simulink model "BugE_v0_40_MAS"  (R2015b)
settings: Solver=FixedStepDiscrete  StartTime=0.0  StopTime=inf  FixedStep=sample_time  RelTol=1e-3
values from neighbouring files (symbols this model uses):
  AB_diode_dV = 0.9    [main_sync.m]
  air_density = 1.225    [main_sync.m]
  bus_charger_Pmax = 1000    [main_sync.m]
  bus_load_Pmax_abs = 500    [main_sync.m]
  capInitVolt = capVmax*sqrt(capInitSoC)    [main_sync.m]
  cyc_kph = [cyc_kph(:,1), cyc_kph(:,2)*speed_max_limit/speed_max]    [main_sync.m]
  cyc_repeat = 0    [main_sync.m]
  ess1_init_soc = 1    [main_sync.m]
  ess1_soh = 1    [main_sync.m]
  ess2_init_soc = 1    [main_sync.m]
  ess2_soh = 1    [main_sync.m]
  ess3_init_soc = 1    [main_sync.m]
  ess3_soh = 1    [main_sync.m]
  ess4_init_soc = 1    [main_sync.m]
  ess4_soh = 1    [main_sync.m]
  ess5_init_soc = 1    [main_sync.m]
  ess5_soh = 1    [main_sync.m]
  gear_ratio = 6    [main_sync.m]
  loadpower = rawcsv(:,2)    [main_sync.m]
  loadtime = rawcsv(:,1)    [main_sync.m]
  lockSOCs = 0    [main_sync.m]
  max_brk_torque = 300    [main_sync.m]
  no_wheels = 3    [main_sync.m]
  period2 = max(loadtime)    [main_sync.m]
  PV_Pmax = 100    [main_sync.m]
  sample_time = 0.01    [main_sync.m]
  startup_seq_step_delay = 0.2    [main_sync.m]
  stop_option = 0    [main_sync.m]
  use_drive_cycle = 1    [main_sync.m]
  use_real_subs_loads = 1    [main_sync.m]
  vbus_max = 25    [main_sync.m]
  vbus_min = 17    [main_sync.m]
  vbus_safety_threshold = 2    [main_sync.m]
  vbus_threshold = 20    [main_sync.m]
  veh_CD = 0.35    [main_sync.m]
  veh_FA = 1.543    [main_sync.m]
  veh_gravity = 9.81*veh_mass    (= 1863.9)    [main_sync.m]
  veh_mass = 190    [main_sync.m]
  wh_1st_rrc = 0.02    [main_sync.m]
  wh_bearing_frc = 0.0015    [main_sync.m]
  wh_inertia = 0.0556    [main_sync.m]
  wh_radius = 0.508/2    (= 0.254)    [main_sync.m]
undefined symbols (not defined in the file or in its folder): capC, capR, cyc_acc, cyc_avg_time_samples, cyc_brk, cyc_grade, cyc_key, DCM_eff_factor_for_Vin, DCM_eff_for_Iout, DCM_Iout, DCM_Iout_max, DCM_Pin_noload, DCM_Pout_max, DCM_Vin, DCM_Vout, DiscIntNeverNeededParam, ess2_coulombic_eff, ess2_Ineg_max_SOC, ess2_Ineg_max_temp, ess2_Ipos_max_SOC, ess2_Ipos_max_temp, ess2_max_ah_cap, ess2_max_volts, ess2_min_volts, ess2_module_parallel, ess2_module_series, ess2_r_dis, ess2_soc, ess2_SOC_for_Ilimit, ess2_temp_for_Ilimit, ess2_temp_max, ess2_tmp, ess2_voc, ess3_coulombic_eff, ess3_max_ah_cap, ess3_module_parallel, ess3_module_series, ess3_r_dis, ess3_soc, ess3_tmp, ess3_voc, ess_coulombic_eff, ess_Ineg_max_SOC, ess_Ineg_max_temp, ess_Ipos_max_SOC, ess_Ipos_max_temp, ess_max_ah_cap, ess_max_volts, ess_min_volts, ess_module_parallel, ess_module_series, ess_nominal_volts, ess_r_dis, ess_soc, ess_SOC_for_Ilimit, ess_temp_for_Ilimit, ess_temp_max, ess_tmp, ess_voc, MC_eff1 ... (+17)
libraries: simulink x139, commfilt2 x1, simulink_extras x1
(part 3 of 7)

== system BugE_v0_40_MAS/Vehicle/Achievable vehicle speed ==
  Vehicle speed at the beginning of the time step [m/s] : Inport
  Available avg. tractive force [N] : Inport  Port=2
  2a : Gain  Gain=2
  4ac : Gain  Gain=4
  Add2 : Sum
  Climbing force : Product  Inputs=3
  Energy Quantification1 : Subsystem
  Gain : Gain  Gain=1/2
  Half the aerodynamic drag at the beginning of the time step : Product
  Product1 : Product
  Saturation : Saturate  UpperLimit=1000  LowerLimit=0
  Tire roll drag force : Product  Inputs=****
  Trig Fn : Trigonometry  Operator=cos
  Trig Fn2 : Trigonometry
  ac : Product  Inputs=**  SaturateOnIntegerOverflow=on  RndMeth=Zero  InputSameDT=on  OutDataTypeStr=Inherit: Same as first input
  aero1 : Constant  Value=0.5*air_density*veh_CD*veh_FA  SampleTime=sample_time
  aero2 : Constant  Value=0.5*air_density*veh_CD*veh_FA  SampleTime=sample_time
  angle of elevation : Trigonometry  Operator=atan
  b^2 : Product  Inputs=**  SaturateOnIntegerOverflow=on  RndMeth=Zero  InputSameDT=on  OutDataTypeStr=Inherit: Same as first input
  delta : Sum  Inputs=+-
  m*v_prev/dt : Product  Inputs=**  SaturateOnIntegerOverflow=on  RndMeth=Zero  InputSameDT=on  OutDataTypeStr=Inherit: Same as first input
  quadratic_a : Gain  Gain=1/2
  quadratic_b : Product  Inputs=*/  SaturateOnIntegerOverflow=on  RndMeth=Zero  InputSameDT=on  OutDataTypeStr=Inherit: Same as first input
  quadratic_c : Sum  Inputs=-++-
  sol : Product  Inputs=/*
  sqrt(delta) : Sqrt  SaturateOnIntegerOverflow=on
  sqrt(delta)-b : Sum  Inputs=-+
  todouble : DataTypeConversion  OutDataTypeStr=double
  u>0 : Fcn  Expr=u>0
  veh_gravity : Constant  Value=veh_gravity  SampleTime=sample_time
  veh_mass : Constant  Value=veh_mass  SampleTime=sample_time
  wh_1st_rrc : Constant  Value=wh_1st_rrc  SampleTime=sample_time
  Vehicle speed at the end of time step [m/s] : Outport
  wires:
  Half the aerodynamic drag at the beginning of the time step/1 -> quadratic_c/2
  Product1/1 -> Gain/1
  aero2/1 -> quadratic_a/1
  Gain/1 -> Half the aerodynamic drag at the beginning of the time step/2
  Add2/1 -> quadratic_c/3
  veh_gravity/1 -> Climbing force/3, Tire roll drag force/4
  Trig Fn/1 -> Tire roll drag force/3
  wh_1st_rrc/1 -> Tire roll drag force/2
  u>0/1 -> Tire roll drag force/1, Climbing force/1
  angle of elevation/1 -> Trig Fn2/1, Trig Fn/1
  m*v_prev/dt/1 -> quadratic_c/1
  [grade] -> angle of elevation/1
  veh_mass/1 -> quadratic_b/1
  aero1/1 -> Half the aerodynamic drag at the beginning of the time step/1
  Trig Fn2/1 -> Climbing force/2
  [dt] -> todouble/1
  Available avg. tractive force [N]/1 -> quadratic_c/4, Energy Quantification1/3(Ftract)
  Tire roll drag force/1 -> Energy Quantification1/1(Froll), Add2/1
  Climbing force/1 -> Energy Quantification1/2(Fclimb), Add2/2
  Vehicle speed at the beginning of the time step [m/s]/1 -> Energy Quantification1/4(Vi), u>0/1, Product1/2, m*v_prev/dt/2, Product1/1
  Saturation/1 -> Vehicle speed at the end of time step [m/s]/1
  quadratic_c/1 -> ac/2
  quadratic_b/1 -> b^2/2, sqrt(delta)-b/1, b^2/1, m*v_prev/dt/1
  ac/1 -> 4ac/1
  4ac/1 -> delta/2
  b^2/1 -> delta/1
  delta/1 -> sqrt(delta)/1
  sqrt(delta)/1 -> sqrt(delta)-b/2
  sqrt(delta)-b/1 -> sol/2
  2a/1 -> sol/1
  quadratic_a/1 -> 2a/1, ac/1
  sol/1 -> Saturation/1
  todouble/1 -> quadratic_b/2

== system BugE_v0_40_MAS/Auxiliaries (LV Grid)/AB (w// diode)/Calculate SOC ==
  Temp [C] : Inport
  I [A] : Inport  Port=2
  1/3600 : Gain  Gain=1/3600
  Add : Sum  Inputs=-+
  Constant1 : Constant  SampleTime=sample_time
  Coulombic efficiency : Lookup_n-D  NumberOfTableDimensions=1  BreakpointsForDimension1=ess3_tmp  Table=ess3_coulombic_eff  InternalRulePriority=Speed  SaturateOnIntegerOverflow=on  InputSameDT=on
  Energy left [Ah] : Sum  Inputs=-+
  I adjusted : Product
  Max capacity [Ah] w/ SOH : Lookup_n-D  NumberOfTableDimensions=1  BreakpointsForDimension1=ess3_tmp  Table=ess3_max_ah_cap*ess5_soh  InternalRulePriority=Speed  SaturateOnIntegerOverflow=on  InputSameDT=on
  Multiply : Product
  Multiply1 : Product
  Resettable Integrator : Subsystem
  "SOC " : Product  Inputs=*/
  Saturation : Saturate  UpperLimit=1  LowerLimit=0
  Switch : Switch  Criteria=u2 > Threshold
  ess2_modules : Constant  Value=ess2_module_series*ess2_module_parallel  SampleTime=sample_time
  SOC : Outport
  wires:
  Resettable Integrator/1(Out1) -> Energy left [Ah]/1
  I [A]/1 -> Switch/2, Switch/1, I adjusted/1
  Switch/1 -> 1/3600/1
  Coulombic efficiency/1 -> I adjusted/2
  Energy left [Ah]/1 -> "SOC "/1
  I adjusted/1 -> Switch/3
  1/3600/1 -> Resettable Integrator/1(input)
  Temp [C]/1 -> Max capacity [Ah] w/ SOH/1, Coulombic efficiency/1
  Multiply1/1 -> Multiply/2, "SOC "/2, Energy left [Ah]/2
  "SOC "/1 -> Saturation/1
  Constant1/1 -> Add/2
  Multiply/1 -> Resettable Integrator/2(IC)
  Add/1 -> Multiply/1
  Saturation/1 -> SOC/1
  ess2_modules/1 -> Multiply1/2
  Max capacity [Ah] w/ SOH/1 -> Multiply1/1
  [AB_SOCinit] -> Add/1

== system BugE_v0_40_MAS/Auxiliaries (LV Grid)/AB (w// diode)/Compute current (nolimit) ==
  Voc [V] : Inport
  Rint [Ohm] : Inport  Port=2
  Output power [W] : Inport  Port=3
  diode_dV [V] : Inport  Port=4
  -b-sqrt(D) : Sum  Inputs=+-
  2*a : Gain  Gain=2
  4*a*c : Gain  Gain=4
  I : Product  Inputs=*/
  I*R : Product  Inputs=**
  Subtract : Sum  Inputs=+-
  Terminator : Terminator
  V_AB : Sum  Inputs=+-
  Voc-Vdiode : Sum  Inputs=+-
  b^2 : Product
  b^2-4*a*c : Sum  Inputs=+-
  c*a : Product
  sqrt(Delta) : Sqrt  SaturateOnIntegerOverflow=on
  I [A] : Outport
  V_out [V] : Outport  Port=2
  wires:
  Output power [W]/1 -> c*a/1
  Voc-Vdiode/1 -> Subtract/1, -b-sqrt(D)/1, b^2/2, b^2/1
  Rint [Ohm]/1 -> c*a/2, 2*a/1, I*R/2
  c*a/1 -> 4*a*c/1
  b^2/1 -> b^2-4*a*c/1
  4*a*c/1 -> b^2-4*a*c/2
  b^2-4*a*c/1 -> sqrt(Delta)/1
  sqrt(Delta)/1 -> -b-sqrt(D)/2
  -b-sqrt(D)/1 -> I/1
  2*a/1 -> I/2
  I/1 -> I [A]/1, I*R/1
  I*R/1 -> Subtract/2, V_AB/2
  Subtract/1 -> V_out [V]/1
  diode_dV [V]/1 -> Voc-Vdiode/2
  Voc [V]/1 -> Voc-Vdiode/1, V_AB/1
  V_AB/1 -> Terminator/1

== system BugE_v0_40_MAS/Auxiliaries (LV Grid)/AB (w// diode)/Energy Quantification ==
  Vout : Inport
  Iout : Inport  Port=2
  R : Inport  Port=3
  diode_dV [V] : Inport  Port=4
  < 0 : Saturate  UpperLimit=0  LowerLimit=-inf
  > 0 : Saturate  UpperLimit=inf  LowerLimit=0  LinearizeAsGain=off
  Diode power : Product
  Gain : Gain  Gain=-1
  P_D+P_R : Sum
  Power : Product
  R power loss : Product  Inputs=3
  tag scope: E_batt_loss5=global, E_batt_regen5=global, E_batt_useful5=global
  wires:
  Vout/1 -> Power/1
  Iout/1 -> Power/2, Diode power/1, R power loss/2, R power loss/1
  Gain/1 -> [E_batt_regen5]
  Power/1 -> < 0/1, > 0/1
  < 0/1 -> Gain/1
  > 0/1 -> [E_batt_useful5]
  R power loss/1 -> P_D+P_R/1
  R/1 -> R power loss/3
  diode_dV [V]/1 -> Diode power/2
  Diode power/1 -> P_D+P_R/2
  P_D+P_R/1 -> [E_batt_loss5]

== system BugE_v0_40_MAS/Auxiliaries (LV Grid)/AB (w// diode)/Pack Voc, R ==
  Temp [degC] : Inport
  SOC_prev : Inport  Port=2
  Req. power [W] : Inport  Port=3
  >=0 : simulink/Logic and Bit Operations/Compare To Zero  relop=>=  OutDataTypeStr=boolean
  Product : Product  Inputs=3
  Product1 : Product  Inputs=/**/
  Product2 : Product  Inputs=/**/
  R_charge [Ohm] : Lookup_n-D  BreakpointsForDimension1=ess2_tmp  BreakpointsForDimension2=ess2_soc  Table=ess2_r_dis  InternalRulePriority=Speed  RndMeth=Simplest  InputSameDT=on
  R_discharge [Ohm] : Lookup_n-D  BreakpointsForDimension1=ess3_tmp  BreakpointsForDimension2=ess3_soc  Table=ess3_r_dis  InternalRulePriority=Speed  RndMeth=Simplest  InputSameDT=on
  Switch : Switch  Criteria=u2 > Threshold
  VOC [V] : Lookup_n-D  BreakpointsForDimension1=ess3_tmp  BreakpointsForDimension2=ess3_soc  Table=ess3_voc  InternalRulePriority=Speed  RndMeth=Simplest  InputSameDT=on
  ess3_module _parallel : Constant  Value=ess3_module_parallel  SampleTime=sample_time
  ess3_module _series : Constant  Value=ess3_module_series  SampleTime=sample_time
  ess5_soh : Constant  Value=ess5_soh  SampleTime=sample_time
  Pack Voc [V] : Outport
  Pack R [Ohm] : Outport  Port=2
  wires:
  Switch/1 -> Pack R [Ohm]/1
  Req. power [W]/1 -> >=0/1
  R_discharge [Ohm]/1 -> Product1/2
  Product/1 -> Pack Voc [V]/1
  VOC [V]/1 -> Product/2
  ess3_module _series/1 -> Product/3, Product2/2, Product1/3
  Temp [degC]/1 -> R_charge [Ohm]/1, R_discharge [Ohm]/1, VOC [V]/1
  SOC_prev/1 -> R_charge [Ohm]/2, R_discharge [Ohm]/2, VOC [V]/2
  ess5_soh/1 -> Product2/1, Product1/1, Product/1
  >=0/1 -> Switch/2
  ess3_module _parallel/1 -> Product1/4, Product2/4
  R_charge [Ohm]/1 -> Product2/3
  Product2/1 -> Switch/3
  Product1/1 -> Switch/1

== system BugE_v0_40_MAS/Auxiliaries (LV Grid)/AB DCDC/Energy Quantification ==
  In1 : Inport
  In2 : Inport  Port=2
  Abs1 : Abs
  Ploss DCM : Sum  Inputs=-+
  tag scope: E_DCM_loss=global
  wires:
  Abs1/1 -> [E_DCM_loss]
  Ploss DCM/1 -> Abs1/1
  In1/1 -> Ploss DCM/1
  In2/1 -> Ploss DCM/2

== system BugE_v0_40_MAS/Auxiliaries (LV Grid)/Auxiliary load/Energy Quantification ==
  Power : Inport
  tag scope: E_accessories=global
  wires:
  Power/1 -> [E_accessories]

== system BugE_v0_40_MAS/Auxiliaries (LV Grid)/ECU & sensors load/Energy Quantification ==
  Power : Inport
  tag scope: E_ECU=global
  wires:
  Power/1 -> [E_ECU]

== system BugE_v0_40_MAS/Energy Storage (New Grid)/AutoPilot/Energy Quantification ==
  Power : Inport
  tag scope: E_autopilot=global
  wires:
  Power/1 -> [E_autopilot]

== system BugE_v0_40_MAS/Energy Storage (New Grid)/Capacitor/Energy Quantification ==
  R : Inport
  Vcap_RC : Inport  Port=2
  Iout : Inport  Port=3
  (I^2)R : Product  Inputs=***
  < 0 : Saturate  UpperLimit=0  LowerLimit=-inf  LinearizeAsGain=off
  > 0 : Saturate  UpperLimit=inf  LowerLimit=0  LinearizeAsGain=off
  Discrete-Time Integrator1 : DiscreteIntegrator  InitialConditionSetting=State (most efficient)  SampleTime=sample_time  ICPrevOutput=DiscIntNeverNeededParam  ICPrevScaledInput=DiscIntNeverNeededParam
  Discrete-Time Integrator2 : DiscreteIntegrator  InitialConditionSetting=State (most efficient)  SampleTime=sample_time  ICPrevOutput=DiscIntNeverNeededParam  ICPrevScaledInput=DiscIntNeverNeededParam
  Display1 : Display
  Display2 : Display
  Gain : Gain  Gain=-1
  Pout_RC1 : Product
  tag scope: E_cap_loss=global, E_cap_regen=global, E_cap_useful=global
  wires:
  Vcap_RC/1 -> Pout_RC1/2
  R/1 -> (I^2)R/1
  > 0/1 -> [E_cap_useful]
  Pout_RC1/1 -> Discrete-Time Integrator2/1, < 0/1, > 0/1
  Iout/1 -> Pout_RC1/1, (I^2)R/2, (I^2)R/3
  (I^2)R/1 -> Discrete-Time Integrator1/1, [E_cap_loss]
  Gain/1 -> [E_cap_regen]
  < 0/1 -> Gain/1
  Discrete-Time Integrator1/1 -> Display1/1  "E cap loss"
  Discrete-Time Integrator2/1 -> Display2/1  "E cap out"

== system BugE_v0_40_MAS/Energy Storage (New Grid)/Charger/Energy Quantification ==
  Power : Inport
  tag scope: E_charger=global
  wires:
  Power/1 -> [E_charger]

== system BugE_v0_40_MAS/Energy Storage (New Grid)/MB1/Calculate SOC ==
  Temp [C] : Inport
  I [A] : Inport  Port=2
  1/3600 : Gain  Gain=1/3600
  Add : Sum  Inputs=-+
  Constant1 : Constant  SampleTime=sample_time
  Coulombic efficiency : Lookup_n-D  NumberOfTableDimensions=1  BreakpointsForDimension1=ess_tmp  Table=ess_coulombic_eff  InternalRulePriority=Speed  SaturateOnIntegerOverflow=on  InputSameDT=on
  Energy left [Ah] : Sum  Inputs=-+
  I adjusted : Product
  Max capacity [Ah] w/ SOH : Lookup_n-D  NumberOfTableDimensions=1  BreakpointsForDimension1=ess_tmp  Table=ess_max_ah_cap*ess1_soh  InternalRulePriority=Speed  SaturateOnIntegerOverflow=on  InputSameDT=on
  Multiply : Product
  Multiply1 : Product
  Resettable Integrator : Subsystem
  "SOC " : Product  Inputs=*/
  Saturation : Saturate  UpperLimit=1  LowerLimit=0
  Switch : Switch  Criteria=u2 > Threshold
  Switch1 : Switch  Criteria=u2 > Threshold
  ess_modules : Constant  Value=ess_module_series*ess_module_parallel  SampleTime=sample_time
  lockSOCs : Constant  Value=lockSOCs
  SOC : Outport
  wires:
  Resettable Integrator/1(Out1) -> Energy left [Ah]/1
  I [A]/1 -> Switch/1, Switch/2, I adjusted/1
  Switch/1 -> 1/3600/1
  Coulombic efficiency/1 -> I adjusted/2
  Energy left [Ah]/1 -> "SOC "/1
  I adjusted/1 -> Switch/3
  1/3600/1 -> Resettable Integrator/1(input)
  Temp [C]/1 -> Max capacity [Ah] w/ SOH/1, Coulombic efficiency/1
  Multiply1/1 -> Multiply/2, "SOC "/2, Energy left [Ah]/2
  "SOC "/1 -> Saturation/1
  [MB1_SOCinit] -> Add/1, Switch1/1
  Constant1/1 -> Add/2
  Multiply/1 -> Resettable Integrator/2(IC)
  Add/1 -> Multiply/1
  Saturation/1 -> Switch1/3
  ess_modules/1 -> Multiply1/2
  Max capacity [Ah] w/ SOH/1 -> Multiply1/1
  lockSOCs/1 -> Switch1/2
  Switch1/1 -> SOC/1

== system BugE_v0_40_MAS/Energy Storage (New Grid)/MB1/Compute current (nolimit) ==
  Voc [V] : Inport
  Rint [Ohm] : Inport  Port=2
  Output power [W] : Inport  Port=3
  2*R : Gain  Gain=2
  4*R*Pbty : Gain  Gain=4
  I*R : Product  Inputs=**
  Ibty : Product  Inputs=*/
  R*Pbty : Product
  Sqrt : Sqrt  SaturateOnIntegerOverflow=on
  "Voc-I*R " : Sum  Inputs=+-
  Voc-sqrt : Sum  Inputs=+-
  Voc^2 : Product
  Voc^2 -4R*Pbty : Sum  Inputs=+-
  I [A] : Outport
  V [V] : Outport  Port=2
  wires:
  Output power [W]/1 -> R*Pbty/1
  Voc [V]/1 -> "Voc-I*R "/1, Voc-sqrt/1, Voc^2/2, Voc^2/1
  Rint [Ohm]/1 -> R*Pbty/2, 2*R/1, I*R/2
  R*Pbty/1 -> 4*R*Pbty/1
  Voc^2/1 -> Voc^2 -4R*Pbty/1
  4*R*Pbty/1 -> Voc^2 -4R*Pbty/2
  Voc^2 -4R*Pbty/1 -> Sqrt/1
  Sqrt/1 -> Voc-sqrt/2
  Voc-sqrt/1 -> Ibty/1
  2*R/1 -> Ibty/2
  Ibty/1 -> I [A]/1, I*R/1
  I*R/1 -> "Voc-I*R "/2
  "Voc-I*R "/1 -> V [V]/1

== system BugE_v0_40_MAS/Energy Storage (New Grid)/MB1/Energy Quantification ==
  V : Inport
  I : Inport  Port=2
  R : Inport  Port=3
  < 0 : Saturate  UpperLimit=0  LowerLimit=-inf
  > 0 : Saturate  UpperLimit=inf  LowerLimit=0  LinearizeAsGain=off
  Gain : Gain  Gain=-1
  Power : Product
  power loss : Product  Inputs=3
  tag scope: E_batt_loss1=global, E_batt_regen1=global, E_batt_useful1=global
  wires:
  V/1 -> Power/1
  I/1 -> Power/2, power loss/2, power loss/1
  Gain/1 -> [E_batt_regen1]
  Power/1 -> < 0/1, > 0/1
  < 0/1 -> Gain/1
  > 0/1 -> [E_batt_useful1]
  power loss/1 -> [E_batt_loss1]
  R/1 -> power loss/3

== system BugE_v0_40_MAS/Energy Storage (New Grid)/MB1/Pack Voc, R ==
  SOC_prev : Inport
  Req. power [W] : Inport  Port=2
  Temp [degC] : Inport  Port=3
  >=0 : simulink/Logic and Bit Operations/Compare To Zero  relop=>=  OutDataTypeStr=boolean
  Constant : Constant  Value=0.9  SampleTime=sample_time
  Constant1 : Constant  SampleTime=sample_time
  Product : Product  Inputs=3
  Product1 : Product  Inputs=/**/
  Product2 : Product  Inputs=/**/
  Product3 : Product
  R_charge [Ohm] : Lookup_n-D  BreakpointsForDimension1=ess_tmp  BreakpointsForDimension2=ess_soc  Table=ess_r_dis  InternalRulePriority=Speed  RndMeth=Simplest  InputSameDT=on
  R_discharge [Ohm] : Lookup_n-D  BreakpointsForDimension1=ess_tmp  BreakpointsForDimension2=ess_soc  Table=ess_r_dis  InternalRulePriority=Speed  RndMeth=Simplest  InputSameDT=on
  Switch : Switch  Criteria=u2 > Threshold
  Switch1 : Switch  Criteria=u2 > Threshold
  VOC [V] : Lookup_n-D  BreakpointsForDimension1=ess_tmp  BreakpointsForDimension2=ess_soc  Table=ess_voc  InternalRulePriority=Speed  RndMeth=Simplest  InputSameDT=on
  ess1_soh : Constant  Value=ess1_soh  SampleTime=sample_time
  ess_module _parallel : Constant  Value=ess_module_parallel  SampleTime=sample_time
  ess_module _series : Constant  Value=ess_module_series  SampleTime=sample_time
  Pack Voc [V] : Outport
  Pack R [Ohm] : Outport  Port=2
  wires:
  Switch/1 -> Pack R [Ohm]/1
  Req. power [W]/1 -> >=0/1
  R_discharge [Ohm]/1 -> Product1/2
  Product/1 -> Pack Voc [V]/1
  VOC [V]/1 -> Product/2
  ess_module _series/1 -> Product/3, Product2/2, Product1/3
  Temp [degC]/1 -> R_charge [Ohm]/1, R_discharge [Ohm]/1, VOC [V]/1
  SOC_prev/1 -> R_charge [Ohm]/2, R_discharge [Ohm]/2, VOC [V]/2
  Product3/1 -> Product2/1, Product1/1, Product/1
  >=0/1 -> Switch/2
  ess_module _parallel/1 -> Product1/4, Product2/4
  R_charge [Ohm]/1 -> Product2/3
  Product2/1 -> Switch/3
  Product1/1 -> Switch/1
  ess1_soh/1 -> Product3/2
  [MB1_lower_SOH] -> Switch1/2
  Constant/1 -> Switch1/1
  Constant1/1 -> Switch1/3
  Switch1/1 -> Product3/1

== system BugE_v0_40_MAS/Energy Storage (New Grid)/MB1 DCDC/Current limiter ==
  enable DCDC : Inport
  I batt side raw : Inport  Port=2
  I bus side raw : Inport  Port=3
  I max : Inport  Port=4
  " ==0 " : simulink/Logic and Bit Operations/Compare To Zero  relop===  OutDataTypeStr=boolean
  0 : Constant  Value=0  SampleTime=sample_time
  ==0 : simulink/Logic and Bit Operations/Compare To Zero  relop===  OutDataTypeStr=boolean
  Abs : Abs
  Abs1 : Abs
  Constant : Constant  SampleTime=sample_time
  Iin final : Product  Inputs=**
  Iin limited : Switch  Criteria=u2 > Threshold
  Iin over limit : RelationalOperator  Operator=>  OutDataTypeStr=boolean
  Iin raw avoid 0 div : Switch  Criteria=u2 > Threshold
  Imax : Product
  Iout final : Product  Inputs=**
  Iout limited : Switch  Criteria=u2 > Threshold
  Iout over limit : RelationalOperator  Operator=<  OutDataTypeStr=boolean
  Iout raw avoid 0 div : Switch  Criteria=u2 > Threshold
  Sign : Signum
  avoid 0 div2 : Switch  Criteria=u2 > Threshold
  avoid 0 div3 : Switch  Criteria=u2 > Threshold
  disable : Logic  Operator=NOT  AllPortsSameDT=off  OutDataTypeStr=boolean
  limit ratio : MinMax  Inputs=2
  limit ratio1 : Product  Inputs=*/
  limit ratio2 : Product  Inputs=*/
  or : Logic  Operator=OR  Inputs=3  AllPortsSameDT=off  OutDataTypeStr=boolean
  I batt side lim : Outport
  I bus side lim : Outport  Port=2
  wires:
  Iout raw avoid 0 div/1 -> Abs1/1, Iout final/2, limit ratio2/2, Iout limited/3
  Iin raw avoid 0 div/1 -> limit ratio1/2, Iin final/1, Iin limited/3, Sign/1, Abs/1
  Iin final/1 -> avoid 0 div2/3
  limit ratio2/1 -> limit ratio/2
  avoid 0 div3/1 -> I bus side lim/1
  Iin over limit/1 -> Iin limited/2
  Iout limited/1 -> limit ratio2/1
  Abs1/1 -> Iout over limit/2
  I max/1 -> Iin over limit/2, Imax/2, Iout over limit/1
  limit ratio/1 -> Iin final/2, Iout final/1
  Imax/1 -> Iin limited/1, Iout limited/1
  Abs/1 -> Iin over limit/1
  Sign/1 -> Imax/1
  limit ratio1/1 -> limit ratio/1
  Iin limited/1 -> limit ratio1/1
  Iout over limit/1 -> Iout limited/2
  I batt side raw/1 -> " ==0 "/1, Iin raw avoid 0 div/3
  enable DCDC/1 -> disable/1
  Constant/1 -> Iout raw avoid 0 div/1, Iin raw avoid 0 div/1
  I bus side raw/1 -> ==0/1, Iout raw avoid 0 div/3
  Iout final/1 -> avoid 0 div3/3
  0/1 -> avoid 0 div2/1, avoid 0 div3/1
  avoid 0 div2/1 -> I batt side lim/1
  or/1 -> avoid 0 div3/2, avoid 0 div2/2, Iin raw avoid 0 div/2, Iout raw avoid 0 div/2
  disable/1 -> or/3
  ==0/1 -> or/2
  " ==0 "/1 -> or/1

== system BugE_v0_40_MAS/Energy Storage (New Grid)/MB1 DCDC/Energy Quantification ==
  In1 : Inport
  In2 : Inport  Port=2
  In3 : Inport  Port=3
  In4 : Inport  Port=4
  Abs : Abs
  P lost : Sum  Inputs=-+
  Pin_DAB : Product
  Pout_DAB : Product
  tag scope: E_DAB1_loss=global
  wires:
  P lost/1 -> Abs/1
  In3/1 -> Pin_DAB/1
  Abs/1 -> [E_DAB1_loss]
  Pin_DAB/1 -> P lost/2
  Pout_DAB/1 -> P lost/1
  In4/1 -> Pin_DAB/2
  In2/1 -> Pout_DAB/2
  In1/1 -> Pout_DAB/1

== system BugE_v0_40_MAS/Energy Storage (New Grid)/MB1 DCDC/eff_maps ==
  "P into bus cmd " : Inport
  Vbus : Inport  Port=2
  Vbatt : Inport  Port=3
  1/V : Product  Inputs=*/
  >= eps : Saturate  UpperLimit=inf  LowerLimit=eps
  Demux : Demux  Outputs=2
  Divide : Product  Inputs=/*
  Gain : Gain  Gain=-1
  Interpolation: efficiency2 : Lookup_n-D  NumberOfTableDimensions=3  BreakpointsForDimension1=MC_Pouts  BreakpointsForDimension2=MC_Vins  BreakpointsForDimension3=MC_Vouts  Table=MC_eff2  InterpMethod=Cubic spline  InternalRulePriority=Speed  RndMeth=Simplest  InputSameDT=on
  Interpolation: efficiency1 : Lookup_n-D  NumberOfTableDimensions=3  BreakpointsForDimension1=MC_Pins  BreakpointsForDimension2=MC_Vins  BreakpointsForDimension3=MC_Vouts  Table=MC_eff1  InterpMethod=Cubic spline  InternalRulePriority=Speed  RndMeth=Simplest  InputSameDT=on
  Mux : Mux  Inputs=2
  Mux1 : Mux  Inputs=2
  Mux2 : Mux  Inputs=2
  P from batt : Switch
  Product : Product
  Saturation : Saturate  UpperLimit=MC_max_eff  LowerLimit=eps
  Saturation1 : Saturate  UpperLimit=MC_max_eff  LowerLimit=eps
  Switch1 : Switch
  I from batt & into bus : Outport
  wires:
  Vbus/1 -> Mux1/2, Mux/1
  Vbatt/1 -> Mux/2, Mux1/1
  Demux/2 -> Interpolation: efficiency1/3, Interpolation: efficiency2/3
  Mux/1 -> Switch1/3
  Switch1/1 -> Demux/1
  Gain/1 -> Interpolation: efficiency1/1
  Interpolation: efficiency2/1 -> Saturation/1
  Divide/1 -> P from batt/1
  Interpolation: efficiency1/1 -> Saturation1/1
  Product/1 -> P from batt/3
  P from batt/1 -> Mux2/1
  "P into bus cmd "/1 -> Gain/1, Interpolation: efficiency2/1, Switch1/2, Divide/2, Product/1, P from batt/2, Mux2/2
  Mux2/1 -> 1/V/1
  Mux1/1 -> >= eps/1, Switch1/1
  1/V/1 -> I from batt & into bus/1
  >= eps/1 -> 1/V/2
  Saturation/1 -> Divide/1
  Saturation1/1 -> Product/2
  Demux/1 -> Interpolation: efficiency2/2, Interpolation: efficiency1/2

== system BugE_v0_40_MAS/Energy Storage (New Grid)/MB1 DCDC/eff_maps1 ==
  I motor : Inport
  Vbatt cmd : Inport  Port=2
  Vbus : Inport  Port=3
  >= eps : Saturate  UpperLimit=inf  LowerLimit=eps
  Gain : Gain  Gain=-1
  I from bus : Product  Inputs=*//
  Interpolation: efficiency2 : Lookup_n-D  NumberOfTableDimensions=3  BreakpointsForDimension1=MC_Pouts  BreakpointsForDimension2=MC_Vins  BreakpointsForDimension3=MC_Vouts  Table=MC_eff2  InterpMethod=Cubic spline  InternalRulePriority=Speed  RndMeth=Simplest  InputSameDT=on
  Mux2 : Mux  Inputs=2
  P out to motor : Product
  Saturation : Saturate  UpperLimit=MC_max_eff  LowerLimit=eps
  I from batt & into bus : Outport
  wires:
  Interpolation: efficiency2/1 -> Saturation/1
  Mux2/1 -> Gain/1
  Gain/1 -> I from batt & into bus/1
  Vbus/1 -> >= eps/1
  Vbatt cmd/1 -> Interpolation: efficiency2/3, P out to motor/2
  I motor/1 -> Mux2/1, P out to motor/1
  P out to motor/1 -> Interpolation: efficiency2/1, I from bus/1
  I from bus/1 -> Mux2/2
  >= eps/1 -> I from bus/3, Interpolation: efficiency2/2
  Saturation/1 -> I from bus/2

== system BugE_v0_40_MAS/Energy Storage (New Grid)/MB2/Calculate SOC ==
  Temp [C] : Inport
  I [A] : Inport  Port=2
  1/3600 : Gain  Gain=1/3600
  Add : Sum  Inputs=-+
  Constant1 : Constant  SampleTime=sample_time
  Coulombic efficiency : Lookup_n-D  NumberOfTableDimensions=1  BreakpointsForDimension1=ess_tmp  Table=ess_coulombic_eff  InternalRulePriority=Speed  SaturateOnIntegerOverflow=on  InputSameDT=on
  Energy left [Ah] : Sum  Inputs=-+
  I adjusted : Product
  Max capacity [Ah] w/ SOH : Lookup_n-D  NumberOfTableDimensions=1  BreakpointsForDimension1=ess_tmp  Table=ess_max_ah_cap*ess2_soh  InternalRulePriority=Speed  SaturateOnIntegerOverflow=on  InputSameDT=on
  Multiply : Product
  Multiply1 : Product
  Resettable Integrator : Subsystem
  "SOC " : Product  Inputs=*/
  Saturation : Saturate  UpperLimit=1  LowerLimit=0
  Switch : Switch  Criteria=u2 > Threshold
  Switch1 : Switch  Criteria=u2 > Threshold
  ess_modules : Constant  Value=ess_module_series*ess_module_parallel  SampleTime=sample_time
  lockSOCs : Constant  Value=lockSOCs
  SOC : Outport
  wires:
  Resettable Integrator/1(Out1) -> Energy left [Ah]/1
  I [A]/1 -> Switch/2, Switch/1, I adjusted/1
  Switch/1 -> 1/3600/1
  Coulombic efficiency/1 -> I adjusted/2
  Energy left [Ah]/1 -> "SOC "/1
  I adjusted/1 -> Switch/3
  1/3600/1 -> Resettable Integrator/1(input)
  Temp [C]/1 -> Max capacity [Ah] w/ SOH/1, Coulombic efficiency/1
  Multiply1/1 -> "SOC "/2, Energy left [Ah]/2, Multiply/2
  "SOC "/1 -> Saturation/1
  Constant1/1 -> Add/2
  Multiply/1 -> Resettable Integrator/2(IC)
  Add/1 -> Multiply/1
  Switch1/1 -> SOC/1
  Max capacity [Ah] w/ SOH/1 -> Multiply1/1
  ess_modules/1 -> Multiply1/2
  [MB2_SOCinit] -> Switch1/1, Add/1
  Saturation/1 -> Switch1/3
  lockSOCs/1 -> Switch1/2

== system BugE_v0_40_MAS/Energy Storage (New Grid)/MB2/Compute current (nolimit) ==
  Voc [V] : Inport
  Rint [Ohm] : Inport  Port=2
  Output power [W] : Inport  Port=3
  2*R : Gain  Gain=2
  4*R*Pbty : Gain  Gain=4
  I*R : Product  Inputs=**
  Ibty : Product  Inputs=*/
  R*Pbty : Product
  Sqrt : Sqrt  SaturateOnIntegerOverflow=on
  "Voc-I*R " : Sum  Inputs=+-
  Voc-sqrt : Sum  Inputs=+-
  Voc^2 : Product
  Voc^2 -4R*Pbty : Sum  Inputs=+-
  I [A] : Outport
  V [V] : Outport  Port=2
  wires:
  Output power [W]/1 -> R*Pbty/1
  Voc [V]/1 -> "Voc-I*R "/1, Voc-sqrt/1, Voc^2/2, Voc^2/1
  Rint [Ohm]/1 -> R*Pbty/2, 2*R/1, I*R/2
  R*Pbty/1 -> 4*R*Pbty/1
  Voc^2/1 -> Voc^2 -4R*Pbty/1
  4*R*Pbty/1 -> Voc^2 -4R*Pbty/2
  Voc^2 -4R*Pbty/1 -> Sqrt/1
  Sqrt/1 -> Voc-sqrt/2
  Voc-sqrt/1 -> Ibty/1
  2*R/1 -> Ibty/2
  Ibty/1 -> I [A]/1, I*R/1
  I*R/1 -> "Voc-I*R "/2
  "Voc-I*R "/1 -> V [V]/1

== system BugE_v0_40_MAS/Energy Storage (New Grid)/MB2/Energy Quantification ==
  In2 : Inport
  In3 : Inport  Port=2
  In1 : Inport  Port=3
  < 0 : Saturate  UpperLimit=0  LowerLimit=-inf
  > 0 : Saturate  UpperLimit=inf  LowerLimit=0  LinearizeAsGain=off
  Gain : Gain  Gain=-1
  Power : Product
  power loss : Product  Inputs=3
  tag scope: E_batt_loss2=global, E_batt_regen2=global, E_batt_useful2=global
  wires:
  In2/1 -> Power/1
  In3/1 -> Power/2, power loss/2, power loss/1
  Gain/1 -> [E_batt_regen2]
  Power/1 -> < 0/1, > 0/1
  < 0/1 -> Gain/1
  > 0/1 -> [E_batt_useful2]
  power loss/1 -> [E_batt_loss2]
  In1/1 -> power loss/3

== system BugE_v0_40_MAS/Energy Storage (New Grid)/MB2/Pack Voc, R ==
  SOC_prev : Inport
  Req. power [W] : Inport  Port=2
  Temp [degC] : Inport  Port=3
  >=0 : simulink/Logic and Bit Operations/Compare To Zero  relop=>=  OutDataTypeStr=boolean
  Product : Product  Inputs=3
  Product1 : Product  Inputs=/**/
  Product2 : Product  Inputs=/**/
  R_charge [Ohm] : Lookup_n-D  BreakpointsForDimension1=ess_tmp  BreakpointsForDimension2=ess_soc  Table=ess_r_dis  InternalRulePriority=Speed  RndMeth=Simplest  InputSameDT=on
  R_discharge [Ohm] : Lookup_n-D  BreakpointsForDimension1=ess_tmp  BreakpointsForDimension2=ess_soc  Table=ess_r_dis  InternalRulePriority=Speed  RndMeth=Simplest  InputSameDT=on
  Switch : Switch  Criteria=u2 > Threshold
  VOC [V] : Lookup_n-D  BreakpointsForDimension1=ess_tmp  BreakpointsForDimension2=ess_soc  Table=ess_voc  InternalRulePriority=Speed  RndMeth=Simplest  InputSameDT=on
  ess2_soh : Constant  Value=ess2_soh  SampleTime=sample_time
  ess_module _parallel : Constant  Value=ess_module_parallel  SampleTime=sample_time
  ess_module _series : Constant  Value=ess_module_series  SampleTime=sample_time
  Pack Voc [V] : Outport
  Pack R [Ohm] : Outport  Port=2
  wires:
  Switch/1 -> Pack R [Ohm]/1
  Req. power [W]/1 -> >=0/1
  R_discharge [Ohm]/1 -> Product1/2
  Product/1 -> Pack Voc [V]/1
  VOC [V]/1 -> Product/2
  ess_module _series/1 -> Product/3, Product2/2, Product1/3
  Temp [degC]/1 -> R_charge [Ohm]/1, R_discharge [Ohm]/1, VOC [V]/1
  SOC_prev/1 -> R_charge [Ohm]/2, R_discharge [Ohm]/2, VOC [V]/2
  ess2_soh/1 -> Product2/1, Product1/1, Product/1
  >=0/1 -> Switch/2
  ess_module _parallel/1 -> Product1/4, Product2/4
  R_charge [Ohm]/1 -> Product2/3
  Product2/1 -> Switch/3
  Product1/1 -> Switch/1

== system BugE_v0_40_MAS/Energy Storage (New Grid)/MB2 DCDC/Current limiter ==
  enable DCDC : Inport
  I batt side raw : Inport  Port=2
  I bus side raw : Inport  Port=3
  I max : Inport  Port=4
  " ==0 " : simulink/Logic and Bit Operations/Compare To Zero  relop===  OutDataTypeStr=boolean
  0 : Constant  Value=0  SampleTime=sample_time
  ==0 : simulink/Logic and Bit Operations/Compare To Zero  relop===  OutDataTypeStr=boolean
  Abs : Abs
  Abs1 : Abs
  Constant : Constant  SampleTime=sample_time
  Iin final : Product  Inputs=**
  Iin limited : Switch  Criteria=u2 > Threshold
  Iin over limit : RelationalOperator  Operator=>  OutDataTypeStr=boolean
  Iin raw avoid 0 div : Switch  Criteria=u2 > Threshold
  Imax : Product
  Iout final : Product  Inputs=**
  Iout limited : Switch  Criteria=u2 > Threshold
  Iout over limit : RelationalOperator  Operator=<  OutDataTypeStr=boolean
  Iout raw avoid 0 div : Switch  Criteria=u2 > Threshold
  Sign : Signum
  avoid 0 div2 : Switch  Criteria=u2 > Threshold
  avoid 0 div3 : Switch  Criteria=u2 > Threshold
  disable : Logic  Operator=NOT  AllPortsSameDT=off  OutDataTypeStr=boolean
  limit ratio : MinMax  Inputs=2
  limit ratio1 : Product  Inputs=*/
  limit ratio2 : Product  Inputs=*/
  or : Logic  Operator=OR  Inputs=3  AllPortsSameDT=off  OutDataTypeStr=boolean
  I batt side lim : Outport
  I bus side lim : Outport  Port=2
  wires:
  Iout raw avoid 0 div/1 -> Abs1/1, Iout final/2, limit ratio2/2, Iout limited/3
  Iin raw avoid 0 div/1 -> limit ratio1/2, Iin final/1, Iin limited/3, Sign/1, Abs/1
  Iin final/1 -> avoid 0 div2/3
  limit ratio2/1 -> limit ratio/2
  avoid 0 div3/1 -> I bus side lim/1
  Iin over limit/1 -> Iin limited/2
  Iout limited/1 -> limit ratio2/1
  Abs1/1 -> Iout over limit/2
  I max/1 -> Iin over limit/2, Imax/2, Iout over limit/1
  limit ratio/1 -> Iin final/2, Iout final/1
  Imax/1 -> Iin limited/1, Iout limited/1
  Abs/1 -> Iin over limit/1
  Sign/1 -> Imax/1
  limit ratio1/1 -> limit ratio/1
  Iin limited/1 -> limit ratio1/1
  Iout over limit/1 -> Iout limited/2
  I batt side raw/1 -> " ==0 "/1, Iin raw avoid 0 div/3
  enable DCDC/1 -> disable/1
  Constant/1 -> Iout raw avoid 0 div/1, Iin raw avoid 0 div/1
  I bus side raw/1 -> ==0/1, Iout raw avoid 0 div/3
  Iout final/1 -> avoid 0 div3/3
  0/1 -> avoid 0 div2/1, avoid 0 div3/1
  avoid 0 div2/1 -> I batt side lim/1
  or/1 -> avoid 0 div3/2, avoid 0 div2/2, Iin raw avoid 0 div/2, Iout raw avoid 0 div/2
  disable/1 -> or/3
  ==0/1 -> or/2
  " ==0 "/1 -> or/1

== system BugE_v0_40_MAS/Energy Storage (New Grid)/MB2 DCDC/Energy Quantification ==
  In1 : Inport
  In2 : Inport  Port=2
  In3 : Inport  Port=3
  In4 : Inport  Port=4
  Abs : Abs
  P lost : Sum  Inputs=-+
  Pin_DAB : Product
  Pout_DAB : Product
  tag scope: E_DAB2_loss=global
  wires:
  P lost/1 -> Abs/1
  In3/1 -> Pin_DAB/1
  Abs/1 -> [E_DAB2_loss]
  Pin_DAB/1 -> P lost/2
  Pout_DAB/1 -> P lost/1
  In4/1 -> Pin_DAB/2
  In2/1 -> Pout_DAB/2
  In1/1 -> Pout_DAB/1

== system BugE_v0_40_MAS/Energy Storage (New Grid)/MB2 DCDC/eff_maps ==
  "P into bus cmd " : Inport
  Vbus : Inport  Port=2
  Vbatt : Inport  Port=3
  1/V : Product  Inputs=*/
  >= eps : Saturate  UpperLimit=inf  LowerLimit=eps
  Clock : Clock
  Demux : Demux  Outputs=2
  Discrete-Time Integrator : DiscreteIntegrator  InitialConditionSetting=State (most efficient)  SampleTime=sample_time  ICPrevOutput=DiscIntNeverNeededParam  ICPrevScaledInput=DiscIntNeverNeededParam
  Discrete-Time Integrator1 : DiscreteIntegrator  InitialConditionSetting=State (most efficient)  SampleTime=sample_time  ICPrevOutput=DiscIntNeverNeededParam  ICPrevScaledInput=DiscIntNeverNeededParam
  Display : Display
  Divide : Product  Inputs=/*
  Divide1 : Product  Inputs=*/
  Gain : Gain  Gain=-1
  Interpolation: efficiency2 : Lookup_n-D  NumberOfTableDimensions=3  BreakpointsForDimension1=MC_Pouts  BreakpointsForDimension2=MC_Vins  BreakpointsForDimension3=MC_Vouts  Table=MC_eff2  InterpMethod=Cubic spline  InternalRulePriority=Speed  RndMeth=Simplest  InputSameDT=on
  Interpolation: efficiency1 : Lookup_n-D  NumberOfTableDimensions=3  BreakpointsForDimension1=MC_Pins  BreakpointsForDimension2=MC_Vins  BreakpointsForDimension3=MC_Vouts  Table=MC_eff1  InterpMethod=Cubic spline  InternalRulePriority=Speed  RndMeth=Simplest  InputSameDT=on
  Mux : Mux  Inputs=2
  Mux1 : Mux  Inputs=2
  Mux2 : Mux  Inputs=2
  P from batt : Switch
  P from batt1 : Switch
  Product : Product
  Saturation : Saturate  UpperLimit=MC_max_eff  LowerLimit=eps
  Saturation1 : Saturate  UpperLimit=MC_max_eff  LowerLimit=eps
  Saturation2 : Saturate  UpperLimit=inf  LowerLimit=eps
  Subtract : Sum  Inputs=+-
  Switch1 : Switch
  avg eff : Display
  I from batt & into bus : Outport
  wires:
  Vbatt/1 -> Mux/2, Mux1/1
  Demux/2 -> Interpolation: efficiency1/3, Interpolation: efficiency2/3
  Mux/1 -> Switch1/3
  Switch1/1 -> Demux/1
  Gain/1 -> Interpolation: efficiency1/1
  Divide/1 -> P from batt/1
  Interpolation: efficiency1/1 -> Saturation1/1
  Product/1 -> P from batt/3
  Mux2/1 -> 1/V/1
  Mux1/1 -> >= eps/1, Switch1/1
  1/V/1 -> I from batt & into bus/1
  >= eps/1 -> 1/V/2
  Demux/1 -> Interpolation: efficiency2/2, Interpolation: efficiency1/2
  Vbus/1 -> Mux1/2, Mux/1
  Saturation/1 -> Divide/1
  P from batt/1 -> Subtract/1, Mux2/1
  Subtract/1 -> Discrete-Time Integrator/1
  Discrete-Time Integrator/1 -> Display/1  "E lost MB2 DCDC"
  Interpolation: efficiency2/1 -> P from batt1/1, Saturation/1
  "P into bus cmd "/1 -> Subtract/2, Gain/1, Interpolation: efficiency2/1, Switch1/2, Divide/2, Product/1, P from batt1/2, P from batt/2, Mux2/2
  Saturation1/1 -> P from batt1/3, Product/2
  P from batt1/1 -> Discrete-Time Integrator1/1
  Discrete-Time Integrator1/1 -> Divide1/1
  Clock/1 -> Saturation2/1
  Divide1/1 -> avg eff/1
  Saturation2/1 -> Divide1/2

== system BugE_v0_40_MAS/Energy Storage (New Grid)/MB2 DCDC/eff_maps1 ==
  I motor : Inport
  Vbatt cmd : Inport  Port=2
  Vbus : Inport  Port=3
  >= eps : Saturate  UpperLimit=inf  LowerLimit=eps
  Gain : Gain  Gain=-1
  I from bus : Product  Inputs=*//
  Interpolation: efficiency2 : Lookup_n-D  NumberOfTableDimensions=3  BreakpointsForDimension1=MC_Pouts  BreakpointsForDimension2=MC_Vins  BreakpointsForDimension3=MC_Vouts  Table=MC_eff2  InterpMethod=Cubic spline  InternalRulePriority=Speed  RndMeth=Simplest  InputSameDT=on
  Mux2 : Mux  Inputs=2
  P out to motor : Product
  Saturation : Saturate  UpperLimit=MC_max_eff  LowerLimit=eps
  I from batt & into bus : Outport
  wires:
  Interpolation: efficiency2/1 -> Saturation/1
  Mux2/1 -> Gain/1
  Gain/1 -> I from batt & into bus/1
  Vbus/1 -> >= eps/1
  Vbatt cmd/1 -> Interpolation: efficiency2/3, P out to motor/2
  I motor/1 -> Mux2/1, P out to motor/1
  P out to motor/1 -> Interpolation: efficiency2/1, I from bus/1
  I from bus/1 -> Mux2/2
  >= eps/1 -> I from bus/3, Interpolation: efficiency2/2
  Saturation/1 -> I from bus/2

== system BugE_v0_40_MAS/Energy Storage (New Grid)/PV_cells Pout/Energy Quantification ==
  Power : Inport
  tag scope: E_PV=global
  wires:
  Power/1 -> [E_PV]

== system BugE_v0_40_MAS/Energy Storage (New Grid)/SB1/Calculate SOC ==
  Temp [C] : Inport
  I [A] : Inport  Port=2
  1/3600 : Gain  Gain=1/3600
  Add : Sum  Inputs=-+
  Constant1 : Constant  SampleTime=sample_time
  Coulombic efficiency : Lookup_n-D  NumberOfTableDimensions=1  BreakpointsForDimension1=ess2_tmp  Table=ess2_coulombic_eff  InternalRulePriority=Speed  SaturateOnIntegerOverflow=on  InputSameDT=on
  Energy used [Ah] : DiscreteIntegrator  InitialConditionSource=external  InitialConditionSetting=State (most efficient)  SampleTime=sample_time  ICPrevOutput=DiscIntNeverNeededParam  ICPrevScaledInput=DiscIntNeverNeededParam
  Energy left [Ah] : Sum  Inputs=-+
  I adjusted : Product
  Max capacity [Ah] w/ SOH : Lookup_n-D  NumberOfTableDimensions=1  BreakpointsForDimension1=ess2_tmp  Table=ess2_max_ah_cap*ess3_soh  InternalRulePriority=Speed  SaturateOnIntegerOverflow=on  InputSameDT=on
  Multiply : Product
  Multiply1 : Product
  "SOC " : Product  Inputs=*/
  Saturation : Saturate  UpperLimit=1  LowerLimit=0
  Switch : Switch  Criteria=u2 > Threshold
  Switch1 : Switch  Criteria=u2 > Threshold
  ess2_modules : Constant  Value=ess2_module_series*ess2_module_parallel  SampleTime=sample_time
  ess3_init_soc : Constant  Value=ess3_init_soc  SampleTime=sample_time
  lockSOCs : Constant  Value=lockSOCs
  SOC : Outport
  wires:
  Energy used [Ah]/1 -> Energy left [Ah]/1
  I [A]/1 -> Switch/2, Switch/1, I adjusted/1
  Switch/1 -> 1/3600/1
  Coulombic efficiency/1 -> I adjusted/2
  Energy left [Ah]/1 -> "SOC "/1
  I adjusted/1 -> Switch/3
  1/3600/1 -> Energy used [Ah]/1
  Temp [C]/1 -> Max capacity [Ah] w/ SOH/1, Coulombic efficiency/1
  Multiply1/1 -> Multiply/2, "SOC "/2, Energy left [Ah]/2
  "SOC "/1 -> Saturation/1
  Constant1/1 -> Add/2
  Multiply/1 -> Energy used [Ah]/2
  Add/1 -> Multiply/1
  ess2_modules/1 -> Multiply1/2
  Max capacity [Ah] w/ SOH/1 -> Multiply1/1
  ess3_init_soc/1 -> Switch1/1, Add/1
  Saturation/1 -> Switch1/3
  lockSOCs/1 -> Switch1/2
  Switch1/1 -> SOC/1

== system BugE_v0_40_MAS/Energy Storage (New Grid)/SB1/Compute current (nolimit) ==
  Voc [V] : Inport
  Rint [Ohm] : Inport  Port=2
  Output power [W] : Inport  Port=3
  2*R : Gain  Gain=2
  4*R*Pbty : Gain  Gain=4
  I*R : Product  Inputs=**
  Ibty : Product  Inputs=*/
  R*Pbty : Product
  Sqrt : Sqrt  SaturateOnIntegerOverflow=on
  "Voc-I*R " : Sum  Inputs=+-
  Voc-sqrt : Sum  Inputs=+-
  Voc^2 : Product
  Voc^2 -4R*Pbty : Sum  Inputs=+-
  I [A] : Outport
  V [V] : Outport  Port=2
  wires:
  Output power [W]/1 -> R*Pbty/1
  Voc [V]/1 -> "Voc-I*R "/1, Voc-sqrt/1, Voc^2/2, Voc^2/1
  Rint [Ohm]/1 -> R*Pbty/2, 2*R/1, I*R/2
  R*Pbty/1 -> 4*R*Pbty/1
  Voc^2/1 -> Voc^2 -4R*Pbty/1
  4*R*Pbty/1 -> Voc^2 -4R*Pbty/2
  Voc^2 -4R*Pbty/1 -> Sqrt/1
  Sqrt/1 -> Voc-sqrt/2
  Voc-sqrt/1 -> Ibty/1
  2*R/1 -> Ibty/2
  Ibty/1 -> I [A]/1, I*R/1
  I*R/1 -> "Voc-I*R "/2
  "Voc-I*R "/1 -> V [V]/1

== system BugE_v0_40_MAS/Energy Storage (New Grid)/SB1/Energy Quantification ==
  In2 : Inport
  In3 : Inport  Port=2
  In1 : Inport  Port=3
  < 0 : Saturate  UpperLimit=0  LowerLimit=-inf
  > 0 : Saturate  UpperLimit=inf  LowerLimit=0  LinearizeAsGain=off
  Gain : Gain  Gain=-1
  Power : Product
  power loss : Product  Inputs=3
  tag scope: E_batt_loss3=global, E_batt_regen3=global, E_batt_useful3=global
  wires:
  In2/1 -> Power/1
  In3/1 -> Power/2, power loss/2, power loss/1
  Gain/1 -> [E_batt_regen3]
  Power/1 -> < 0/1, > 0/1
  < 0/1 -> Gain/1
  > 0/1 -> [E_batt_useful3]
  power loss/1 -> [E_batt_loss3]
  In1/1 -> power loss/3

== system BugE_v0_40_MAS/Energy Storage (New Grid)/SB1/Pack Voc, R ==
  SOC_prev : Inport
  Req. power [W] : Inport  Port=2
  Temp [degC] : Inport  Port=3
  >=0 : simulink/Logic and Bit Operations/Compare To Zero  relop=>=  OutDataTypeStr=boolean
  Product : Product  Inputs=3
  Product1 : Product  Inputs=/**/
  Product2 : Product  Inputs=/**/
  R_charge [Ohm] : Lookup_n-D  BreakpointsForDimension1=ess2_tmp  BreakpointsForDimension2=ess2_soc  Table=ess2_r_dis  InternalRulePriority=Speed  RndMeth=Simplest  InputSameDT=on
  R_discharge [Ohm] : Lookup_n-D  BreakpointsForDimension1=ess2_tmp  BreakpointsForDimension2=ess2_soc  Table=ess2_r_dis  InternalRulePriority=Speed  RndMeth=Simplest  InputSameDT=on
  Switch : Switch  Criteria=u2 > Threshold
  VOC [V] : Lookup_n-D  BreakpointsForDimension1=ess2_tmp  BreakpointsForDimension2=ess2_soc  Table=ess2_voc  InternalRulePriority=Speed  RndMeth=Simplest  InputSameDT=on
  ess2_module _parallel : Constant  Value=ess2_module_parallel  SampleTime=sample_time
  ess2_module _series : Constant  Value=ess2_module_series  SampleTime=sample_time
  ess3_soh : Constant  Value=ess3_soh  SampleTime=sample_time
  Pack Voc [V] : Outport
  Pack R [Ohm] : Outport  Port=2
  wires:
  Switch/1 -> Pack R [Ohm]/1
  Req. power [W]/1 -> >=0/1
  R_discharge [Ohm]/1 -> Product1/2
  Product/1 -> Pack Voc [V]/1
  VOC [V]/1 -> Product/2
  ess2_module _series/1 -> Product/3, Product2/2, Product1/3
  Temp [degC]/1 -> R_charge [Ohm]/1, R_discharge [Ohm]/1, VOC [V]/1
  SOC_prev/1 -> R_charge [Ohm]/2, R_discharge [Ohm]/2, VOC [V]/2
  ess3_soh/1 -> Product2/1, Product1/1, Product/1
  >=0/1 -> Switch/2
  ess2_module _parallel/1 -> Product1/4, Product2/4
  R_charge [Ohm]/1 -> Product2/3
  Product2/1 -> Switch/3
  Product1/1 -> Switch/1

== system BugE_v0_40_MAS/Energy Storage (New Grid)/SB1 DCDC/Current limiter ==
  enable DCDC : Inport
  I batt side raw : Inport  Port=2
  I bus side raw : Inport  Port=3
  I max : Inport  Port=4
  " ==0 " : simulink/Logic and Bit Operations/Compare To Zero  relop===  OutDataTypeStr=boolean
  0 : Constant  Value=0  SampleTime=sample_time
  ==0 : simulink/Logic and Bit Operations/Compare To Zero  relop===  OutDataTypeStr=boolean
  Abs : Abs
  Abs1 : Abs
  Constant : Constant  SampleTime=sample_time
  Iin final : Product  Inputs=**
  Iin limited : Switch  Criteria=u2 > Threshold
  Iin over limit : RelationalOperator  Operator=>  OutDataTypeStr=boolean
  Iin raw avoid 0 div : Switch  Criteria=u2 > Threshold
  Imax : Product
  Iout final : Product  Inputs=**
  Iout limited : Switch  Criteria=u2 > Threshold
  Iout over limit : RelationalOperator  Operator=<  OutDataTypeStr=boolean
  Iout raw avoid 0 div : Switch  Criteria=u2 > Threshold
  Sign : Signum
  avoid 0 div2 : Switch  Criteria=u2 > Threshold
  avoid 0 div3 : Switch  Criteria=u2 > Threshold
  disable : Logic  Operator=NOT  AllPortsSameDT=off  OutDataTypeStr=boolean
  limit ratio : MinMax  Inputs=2
  limit ratio1 : Product  Inputs=*/
  limit ratio2 : Product  Inputs=*/
  or : Logic  Operator=OR  Inputs=3  AllPortsSameDT=off  OutDataTypeStr=boolean
  I batt side lim : Outport
  I bus side lim : Outport  Port=2
  wires:
  Iout raw avoid 0 div/1 -> Abs1/1, Iout final/2, limit ratio2/2, Iout limited/3
  Iin raw avoid 0 div/1 -> limit ratio1/2, Iin final/1, Iin limited/3, Sign/1, Abs/1
  Iin final/1 -> avoid 0 div2/3
  limit ratio2/1 -> limit ratio/2
  avoid 0 div3/1 -> I bus side lim/1
  Iin over limit/1 -> Iin limited/2
  Iout limited/1 -> limit ratio2/1
  Abs1/1 -> Iout over limit/2
  I max/1 -> Iin over limit/2, Imax/2, Iout over limit/1
  limit ratio/1 -> Iin final/2, Iout final/1
  Imax/1 -> Iin limited/1, Iout limited/1
  Abs/1 -> Iin over limit/1
  Sign/1 -> Imax/1
  limit ratio1/1 -> limit ratio/1
  Iin limited/1 -> limit ratio1/1
  Iout over limit/1 -> Iout limited/2
  I batt side raw/1 -> " ==0 "/1, Iin raw avoid 0 div/3
  enable DCDC/1 -> disable/1
  Constant/1 -> Iout raw avoid 0 div/1, Iin raw avoid 0 div/1
  I bus side raw/1 -> ==0/1, Iout raw avoid 0 div/3
  Iout final/1 -> avoid 0 div3/3
  0/1 -> avoid 0 div2/1, avoid 0 div3/1
  avoid 0 div2/1 -> I batt side lim/1
  or/1 -> avoid 0 div3/2, avoid 0 div2/2, Iin raw avoid 0 div/2, Iout raw avoid 0 div/2
  disable/1 -> or/3
  ==0/1 -> or/2
  " ==0 "/1 -> or/1

== system BugE_v0_40_MAS/Energy Storage (New Grid)/SB1 DCDC/Energy Quantification ==
  In1 : Inport
  In2 : Inport  Port=2
  In3 : Inport  Port=3
  In4 : Inport  Port=4
  Abs : Abs
  P lost : Sum  Inputs=-+
  Pin_DAB : Product
  Pout_DAB : Product
  tag scope: E_DAB3_loss=global
  wires:
  P lost/1 -> Abs/1
  In3/1 -> Pin_DAB/1
  Abs/1 -> [E_DAB3_loss]
  Pin_DAB/1 -> P lost/2
  Pout_DAB/1 -> P lost/1
  In4/1 -> Pin_DAB/2
  In2/1 -> Pout_DAB/2
  In1/1 -> Pout_DAB/1

== system BugE_v0_40_MAS/Energy Storage (New Grid)/SB1 DCDC/eff_maps1 ==
  "P into bus cmd " : Inport
  Vbus : Inport  Port=2
  Vbatt : Inport  Port=3
  1/V : Product  Inputs=*/
  >= eps : Saturate  UpperLimit=inf  LowerLimit=eps
  Demux : Demux  Outputs=2
  Divide : Product  Inputs=/*
  Gain : Gain  Gain=-1
  Interpolation: efficiency2 : Lookup_n-D  NumberOfTableDimensions=3  BreakpointsForDimension1=MC_Pouts  BreakpointsForDimension2=MC_Vins  BreakpointsForDimension3=MC_Vouts  Table=MC_eff2  InterpMethod=Cubic spline  InternalRulePriority=Speed  RndMeth=Simplest  InputSameDT=on
  Interpolation: efficiency1 : Lookup_n-D  NumberOfTableDimensions=3  BreakpointsForDimension1=MC_Pins  BreakpointsForDimension2=MC_Vins  BreakpointsForDimension3=MC_Vouts  Table=MC_eff1  InterpMethod=Cubic spline  InternalRulePriority=Speed  RndMeth=Simplest  InputSameDT=on
  Mux : Mux  Inputs=2
  Mux1 : Mux  Inputs=2
  Mux2 : Mux  Inputs=2
  P from batt : Switch
  Product : Product
  Saturation : Saturate  UpperLimit=MC_max_eff  LowerLimit=eps
  Saturation1 : Saturate  UpperLimit=MC_max_eff  LowerLimit=eps
  Switch1 : Switch
  I from batt & into bus : Outport
  wires:
  Vbus/1 -> Mux1/2, Mux/1
  Vbatt/1 -> Mux/2, Mux1/1
  Demux/2 -> Interpolation: efficiency1/3, Interpolation: efficiency2/3
  Mux/1 -> Switch1/3
  Switch1/1 -> Demux/1
  Gain/1 -> Interpolation: efficiency1/1
  Interpolation: efficiency2/1 -> Saturation/1
  Divide/1 -> P from batt/1
  Interpolation: efficiency1/1 -> Saturation1/1
  Product/1 -> P from batt/3
  P from batt/1 -> Mux2/1
  "P into bus cmd "/1 -> Gain/1, Interpolation: efficiency2/1, Switch1/2, Divide/2, Product/1, P from batt/2, Mux2/2
  Mux2/1 -> 1/V/1
  Mux1/1 -> >= eps/1, Switch1/1
  1/V/1 -> I from batt & into bus/1
  >= eps/1 -> 1/V/2
  Saturation/1 -> Divide/1
  Saturation1/1 -> Product/2
  Demux/1 -> Interpolation: efficiency2/2, Interpolation: efficiency1/2

== system BugE_v0_40_MAS/Energy Storage (New Grid)/SB2/Calculate SOC ==
  Temp [C] : Inport
  I [A] : Inport  Port=2
  1/3600 : Gain  Gain=1/3600
  Add : Sum  Inputs=-+
  Constant1 : Constant  SampleTime=sample_time
  Coulombic efficiency : Lookup_n-D  NumberOfTableDimensions=1  BreakpointsForDimension1=ess2_tmp  Table=ess2_coulombic_eff  InternalRulePriority=Speed  SaturateOnIntegerOverflow=on  InputSameDT=on
  Energy used [Ah] : DiscreteIntegrator  InitialConditionSource=external  InitialConditionSetting=State (most efficient)  SampleTime=sample_time  ICPrevOutput=DiscIntNeverNeededParam  ICPrevScaledInput=DiscIntNeverNeededParam
  Energy left [Ah] : Sum  Inputs=-+
  I adjusted : Product
  Max capacity [Ah] w/ SOH : Lookup_n-D  NumberOfTableDimensions=1  BreakpointsForDimension1=ess2_tmp  Table=ess2_max_ah_cap*ess4_soh  InternalRulePriority=Speed  SaturateOnIntegerOverflow=on  InputSameDT=on
  Multiply : Product
  Multiply1 : Product
  "SOC " : Product  Inputs=*/
  Saturation : Saturate  UpperLimit=1  LowerLimit=0
  Switch : Switch  Criteria=u2 > Threshold
  Switch1 : Switch  Criteria=u2 > Threshold
  ess2_modules : Constant  Value=ess2_module_series*ess2_module_parallel  SampleTime=sample_time
  ess3_init_soc : Constant  Value=ess4_init_soc  SampleTime=sample_time
  lockSOCs : Constant  Value=lockSOCs
  SOC : Outport
  wires:
  Energy used [Ah]/1 -> Energy left [Ah]/1
  I [A]/1 -> Switch/2, Switch/1, I adjusted/1
  Switch/1 -> 1/3600/1
  Coulombic efficiency/1 -> I adjusted/2
  Energy left [Ah]/1 -> "SOC "/1
  I adjusted/1 -> Switch/3
  1/3600/1 -> Energy used [Ah]/1
  Temp [C]/1 -> Max capacity [Ah] w/ SOH/1, Coulombic efficiency/1
  Multiply1/1 -> Multiply/2, "SOC "/2, Energy left [Ah]/2
  "SOC "/1 -> Saturation/1
  Constant1/1 -> Add/2
  Multiply/1 -> Energy used [Ah]/2
  Add/1 -> Multiply/1
  ess2_modules/1 -> Multiply1/2
  Max capacity [Ah] w/ SOH/1 -> Multiply1/1
  ess3_init_soc/1 -> Switch1/1, Add/1
  Saturation/1 -> Switch1/3
  lockSOCs/1 -> Switch1/2
  Switch1/1 -> SOC/1
